simulink model "UnitTest_relay_model"  (Simulink 8.1)
settings: Solver=ode1  StartTime=0.0  StopTime=inf  FixedStep=Ts  MaxStep=1e-3  RelTol=1e-3
model workspace (MAT data in the model file):
  op_snapshot1 : opcond.OperatingPoint (value not decoded)
PostLoadFcn:
  | UnitTest_relay_model_init;
InitFcn:
  | UnitTest_relay_model_init;
values from neighbouring files (symbols this model uses):
  relay_par = xlsread('relay_parameters.xlsx')    [relay_settings_init.m]
undefined symbols (not defined in the file or in its folder): Ts
libraries: powerlib x3, rtlab x2, cables_lib x2, breaker_lib x2, artemis x1, simulink x1, relay_modbus_lib x1, rtio_generic_modbus x1, Load_lib x1, transformer_lib x1
settings Model: ARTEMISmethode_block_infos=$$__separator__$$UnitTest_relay_model/ARTEMIS Guide$$__separator__$$  Creator=RE25624  LastModifiedBy=re25624  BufferReuse=off
settings SolverCC: ZeroCrossAlgorithm=Adaptive
settings DataIOCC: ExternalInput=getinputstruct(op_snapshot1)  InitialState=getstatestruct(op_snapshot1)  LimitDataPoints=off  MaxDataPoints=90060  SignalLoggingSaveFormat=Dataset  SaveOutput=off  SignalLogging=off  DSMLogging=off  SaveTime=off  OutputSaveName=result
settings OptimizationCC: BlockReduction=off  OptimizeBlockIOStorage=off  BufferReuse=off  ExpressionFolding=off  LocalBlockOutputs=off
settings DebuggingCC: MaxConsecutiveZCsMsg=warning  IgnoredZcDiagnostic=none  SolverPrmCheckMsg=none  MultiTaskRateTransMsg=warning  FcnCallInpInsideContextMsg=EnableAllAsWarning  FrameProcessingCompatibilityMsg=error  ModelReferenceExtraNoncontSigs=warning  StrictBusMsg=None
settings ModelReferenceCC: UpdateModelReferenceTargets=IfOutOfDate
settings SFSimCC: SFSimEcho=off
settings GRTTargetCC: CodeReplacementLibrary=C89/C90 (ANSI)

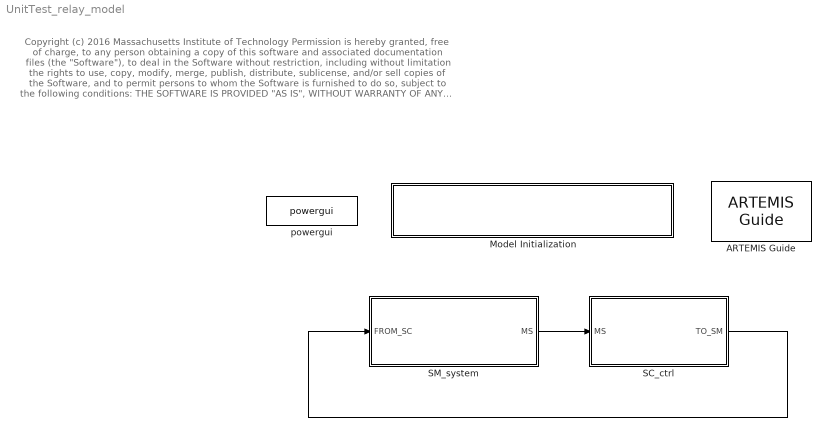
== system UnitTest_relay_model ==
  note: Copyright (c) 2016 Massachusetts Institute of Technology
      | Permission is hereby granted, free of charge, to any person obtaining a copy of this software and associated documentation files (the "Software"), to deal
      | in the Software without restriction, including without limitation the rights to use, copy, modify, merge, publish, distribute, sublicense, and/or sell copies of the
      | Software, and to permit persons to whom the Software is furnished to do so, subject to the following conditions:
      |
      | THE SOFTWARE IS PROVIDED "AS IS", WITHOUT WARRANTY OF ANY KIND, EXPRESS OR IMPLIED, INCLUDING BUT NOT LIMITED TO THE
      | WARRANTIES OF MERCHANTABILITY, FITNESS FOR A PARTICULAR PURPOSE AND NONINFRINGEMENT. IN NO EVENT SHALL THE AUTHORS
      | OR COPYRIGHT HOLDERS BE LIABLE FOR ANY CLAIM, DAMAGES OR OTHER LIABILITY, WHETHER IN AN ACTION OF CONTRACT, TORT OR
      | OTHERWISE, ARISING FROM, OUT OF OR IN CONNECTION WITH THE SOFTWARE OR THE USE OR OTHER DEALINGS IN THE SOFTWARE.
  ARTEMIS Guide : artemis/ARTEMIS/ARTEMIS Guide  Tag=FTSSmethode_opal_4hx0r99  Description=5.0_z1  lock=on  Ts=Ts  opt=art5  dyna=off  nb_perm=4  RT_fullcomp=off  ssn=on  ssn_itvc=off  ssn_ivic=off  ssn_ext=off  ssn_solver=Art5 with Backward Euler nodal interface  ssn_impulse=off  ssn_quasimpulse=off  ssn_impulse_loop=2  paraExtinctionThy=off  Thy_Impulse=on  dtc=Off  dtc_opt=normal  ao=on  simtype=off  ct_mac=off  lin_mov=off  lsp=[0.001 2]  spike_skip=Disabled  dtc_extra=1  dtc_sws=normal  dtc_pied=0.5  SPSRulesBlock=SPSRules  tre=on  ctmm=off  LF=off  dpl_type=ARTEMiS DPL  rlc_type=off  custom_type=off  para=on  ssn_ImpulseLoopBlockedStateUpdate=2  ssn_mov_iter_number=5  ssn_switch_iter_number=5
  Model Initialization : Subsystem  AncestorBlock=artemis/Tools /Misc/Model Initialization  mask(Model Functions){InitFcnX=UnitTest_relay_model_init;, prel=off, posl=on, inif=on, strf=off}
      mask prompts: InitFcnX "Initialisation"; prel "Preload Function"; posl "PostLoad Function"; inif "InitFcn"; strf "StartFcn"
      mask init:
      | currentBlock = gcb;
      | root = bdroot(currentBlock);
      | 
      | 
      | if ~strcmp(get_param(root,'BlockDiagramType'),'library')
      |     if prel==1
      |         set_param(root, 'PreLoadFcn', InitFcnX);
      |     else
      |         set_param(root, 'PreLoadFcn', '');
      |     end
      |     if inif==1
      |         set_param(root, 'InitFcn', InitFcnX);
      |     else
      |         set_param(root, 'InitFcn', '');
      |     end
      |     if strf==1
      |         set_param(root, 'StartFcn', InitFcnX);
      |     else
      |         set_param(root, 'StartFcn', '');
      |     end
      |     if posl==1
      |         set_param(root, 'PostLoadFcn', InitFcnX);
      |     else
      |         set_param(root, 'PostLoadFcn', '');
      |     end
      | end
      | 
      | pos = get_param(currentBlock, 'Position');
      | width = pos(3) - pos(1); height = pos(4) - pos(2);
      | txt = [ upper(root) '\n' '- InitFcn. . . . . '  get_param(root, 'InitFcn') ];
      settings: CopyFcn=set_param(gcb,'LinkStatus','inactive')
      mask Display: text(5, height*0.5, txt, 'horizontalAlignment', 'left', 'verticalAlignment', 'middle') ;
  SC_ctrl : Subsystem
  SM_system : Subsystem
  powergui : powerlib/powergui  Priority=2  SimulationMode=Discrete  SolverType=Tustin  SampleTime=Ts  frequency=60  SPID=off  DisableSnubberDevices=off  DisableRonSwitches=off  DisableVfSwitches=off  SwTol=0  Interpol=off  DisplayEquations=off  frequencyindice=0  Pbase=100e6  ErrMax=1e-4  Iterations=50  UnitsV=kV  UnitsW=MW  FunctionMessages=off  echomessages=off  HookPort=off  EnableUseOfTLC=off  x0status=blocks  RestoreLinks=warning  ResistiveCurrentMeasurement=off  Frange=logspace(0,3,50)  Ylog=off  Xlog=off  ShowGrid=off  save=off  variable=ZData  structure=0  ZoomFFT=on  StartTime=0.0  cycles=2  DisplayStyle=off  fundamental=60  FreqAxis=off  MaxFrequency=1000  frequencyindicesteady=1  RmsSteady=1  display=off  Ts=0  methode=off
  wires:
  SM_system/1(MS) -> SC_ctrl/1(MS)
  SC_ctrl/1(TO_SM) -> SM_system/1(FROM_SC)

== system UnitTest_relay_model/Model Initialization ==

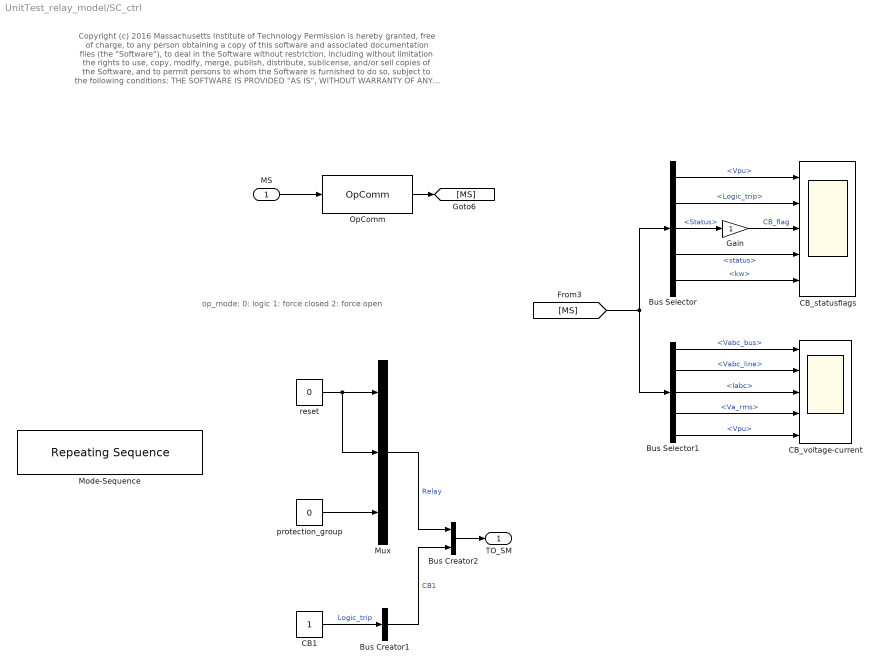
== system UnitTest_relay_model/SC_ctrl ==
  note: op_mode:
      | 0: logic
      | 1: force closed
      | 2: force open
  note: Copyright (c) 2016 Massachusetts Institute of Technology
      | Permission is hereby granted, free of charge, to any person obtaining a copy of this software and associated documentation files (the "Software"), to deal
      | in the Software without restriction, including without limitation the rights to use, copy, modify, merge, publish, distribute, sublicense, and/or sell copies of the
      | Software, and to permit persons to whom the Software is furnished to do so, subject to the following conditions:
      |
      | THE SOFTWARE IS PROVIDED "AS IS", WITHOUT WARRANTY OF ANY KIND, EXPRESS OR IMPLIED, INCLUDING BUT NOT LIMITED TO THE
      | WARRANTIES OF MERCHANTABILITY, FITNESS FOR A PARTICULAR PURPOSE AND NONINFRINGEMENT. IN NO EVENT SHALL THE AUTHORS
      | OR COPYRIGHT HOLDERS BE LIABLE FOR ANY CLAIM, DAMAGES OR OTHER LIABILITY, WHETHER IN AN ACTION OF CONTRACT, TORT OR
      | OTHERWISE, ARISING FROM, OUT OF OR IN CONNECTION WITH THE SOFTWARE OR THE USE OR OTHER DEALINGS IN THE SOFTWARE
  MS : Inport
  Bus Creator1 : BusCreator  Inputs=1
  Bus Creator2 : BusCreator  Inputs=2
  Bus Selector : BusSelector  OutputSignals=relay_cmd.m.Vpu,relay_cmd.Logic_trip,CB.Status,relay_cmd.m.status,relay_cmd.m.kw
  Bus Selector1 : BusSelector  OutputSignals=CB.Vabc_bus,CB.Vabc_line,CB.Iabc,relay_cmd.m.Va_rms,relay_cmd.m.Vpu
  CB1 : Constant
  CB_statusflags : Scope  NumInputPorts=5
      settings: ShowLegends=on  TimeRange=0.35  YMin=-0.01~-0.5~0~0~0  YMax=0.01~3~2~10~2500  SaveName=ScopeData6
  CB_voltage-current : Scope  NumInputPorts=5
      settings: ShowLegends=on  TimeRange=3  YMin=-12500~-12500~-175~0~0  YMax=12500~12500~175~10000~1.2
  Gain : Gain
  Mode-Sequence : simulink/Sources/Repeating Sequence  rep_seq_t=|  rep_seq_y=|
      rep_seq_t=|
      | [0
      | 2
      | 2
      | 4
      | 4
      | 6
      | 6
      | 8
      | 8
      | 10
      | 10
      | 12
      | 12
      | 14
      | 14
      | 16]
      rep_seq_y=|
      | [0
      | 0
      | 1
      | 1
      | 0
      | 0
      | 2
      | 2
      | 1
      | 1
      | 0
      | 0
      | 2
      | 2
      | 0
      | 0]
  Mux : Mux  Inputs=3
  OpComm : rtlab/OpComm  nbport=1  groupe_acq=1  subsys_rate=0  st=0  Synchronization=on  Interpolation=on  Threshold=1.0  Missed_Data=off  Sim_Time=off  Samples=off  dynSigOut=off  from_console=0  warning_done=off  writeOpCommFile=off  Offset=off
  protection_group : Constant  Value=0
  reset : Constant  Value=0
  TO_SM : Outport
  wires:
  OpComm/1 -> [MS]
  MS/1 -> OpComm/1
  [MS] -> Bus Selector/1, Bus Selector1/1
  Bus Selector/5 -> CB_statusflags/5  "<kw>"
  Bus Selector/1 -> CB_statusflags/1  "<Vpu>"
  Bus Selector/2 -> CB_statusflags/2  "<Logic_trip>"
  Bus Selector/4 -> CB_statusflags/4  "<status>"
  Bus Selector/3 -> Gain/1  "<Status>"
  Gain/1 -> CB_statusflags/3  "CB_flag"
  Bus Selector1/2 -> CB_voltage-current/2  "<Vabc_line>"
  Bus Selector1/1 -> CB_voltage-current/1  "<Vabc_bus>"
  Bus Selector1/3 -> CB_voltage-current/3  "<Iabc>"
  Mux/1 -> Bus Creator2/1  "Relay"
  reset/1 -> Mux/2, Mux/1
  protection_group/1 -> Mux/3
  Bus Selector1/4 -> CB_voltage-current/4  "<Va_rms>"
  Bus Selector1/5 -> CB_voltage-current/5  "<Vpu>"
  CB1/1 -> Bus Creator1/1  "Logic_trip"
  Bus Creator1/1 -> Bus Creator2/2  "CB1"
  Bus Creator2/1 -> TO_SM/1

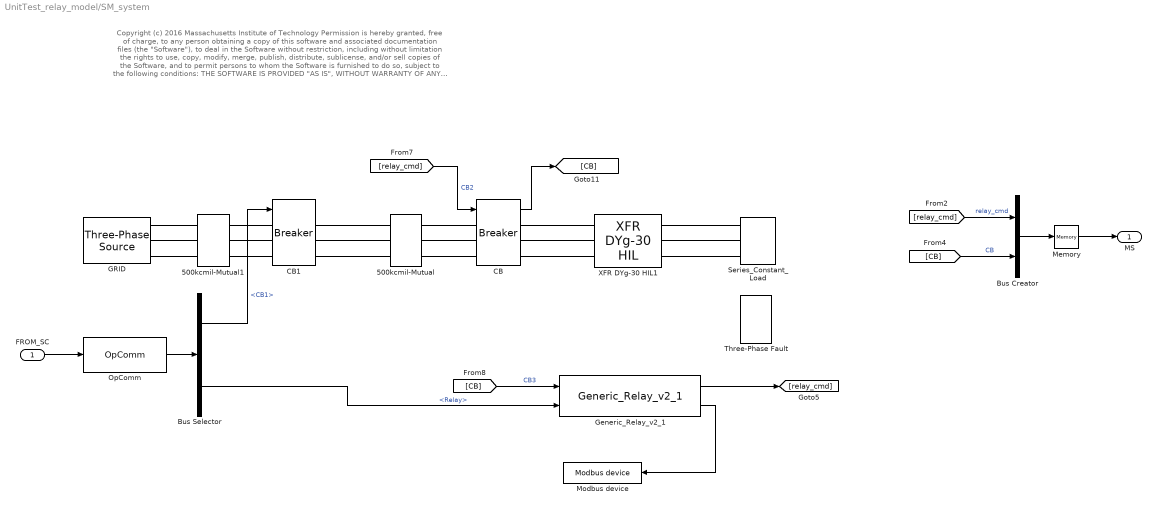
== system UnitTest_relay_model/SM_system ==
  note: Copyright (c) 2016 Massachusetts Institute of Technology
      | Permission is hereby granted, free of charge, to any person obtaining a copy of this software and associated documentation files (the "Software"), to deal
      | in the Software without restriction, including without limitation the rights to use, copy, modify, merge, publish, distribute, sublicense, and/or sell copies of the
      | Software, and to permit persons to whom the Software is furnished to do so, subject to the following conditions:
      |
      | THE SOFTWARE IS PROVIDED "AS IS", WITHOUT WARRANTY OF ANY KIND, EXPRESS OR IMPLIED, INCLUDING BUT NOT LIMITED TO THE
      | WARRANTIES OF MERCHANTABILITY, FITNESS FOR A PARTICULAR PURPOSE AND NONINFRINGEMENT. IN NO EVENT SHALL THE AUTHORS
      | OR COPYRIGHT HOLDERS BE LIABLE FOR ANY CLAIM, DAMAGES OR OTHER LIABILITY, WHETHER IN AN ACTION OF CONTRACT, TORT OR
      | OTHERWISE, ARISING FROM, OUT OF OR IN CONNECTION WITH THE SOFTWARE OR THE USE OR OTHER DEALINGS IN THE SOFTWARE
  FROM_SC : Inport
  500kcmil-Mutual : cables_lib/500kcmil-Mutual  length=1100  par_sets=1  ratio=3
  500kcmil-Mutual1 : cables_lib/500kcmil-Mutual  length=1100  par_sets=1  ratio=3
  Bus Creator : BusCreator  Inputs=2
  Bus Selector : BusSelector  OutputSignals=CB1,Relay
  CB : breaker_lib/Breaker  Ts=Ts  mech_delay=cb_mech_delay
  CB1 : breaker_lib/Breaker  Ts=Ts  mech_delay=cb_mech_delay
  GRID : powerlib/Electrical Sources/Three-Phase Source  Voltage=13800  PhaseAngle=0  Frequency=60  InternalConnection=Yg  SpecifyImpedance=on  Resistance=0.8929  Inductance=16.58e-3  ShortCircuitLevel=375e6  BaseVoltage=13800  XRratio=30  BusType=swing  Pref=0  Qref=0  Qmin=-inf  Qmax=inf
  Generic_Relay_v2_1 : relay_modbus_lib/Generic_Relay_v2_1  Ts=Ts  relay_settings=[relay_par(1,:)]
  Memory : Memory
  Modbus device : rtio_generic_modbus/Modbus device  conf_name=F1_relay_cfg2.opal  conf_name_mask=F1_relay_cfg2.xls  sample_time=Ts
  OpComm : rtlab/OpComm  nbport=1  groupe_acq=1  subsys_rate=0  st=0  Synchronization=on  Interpolation=on  Threshold=1.0  Missed_Data=off  Sim_Time=off  Samples=off  dynSigOut=off  from_console=1  warning_done=off  writeOpCommFile=off  Offset=off
  Series_Constant_Load : Load_lib/Series_Constant_Load  v=460  kVA=2500  pf=0.90
  Three-Phase Fault : powerlib/Elements/Three-Phase Fault  FaultA=on  FaultB=on  FaultC=on  FaultResistance=0.001  GroundFault=on  GroundResistance=0.001  External=off  SwitchStatus=[1 0]  SwitchTimes=[ 2.2 9]  InitialStates=[0 0 1]  SnubberResistance=1e6  SnubberCapacitance=inf  Measurements=None
  XFR DYg-30 HIL1 : transformer_lib/XFR DYg-30 HIL  Rating=2500  Vp=13800  Vs=480  Z=5.75  XR=6.6
  MS : Outport
  wires:
  CB/1 -> [CB]
  Bus Creator/1 -> Memory/1
  [relay_cmd] -> Bus Creator/1  "relay_cmd"
  [CB] -> Bus Creator/2  "CB"
  Memory/1 -> MS/1
  [CB] -> Generic_Relay_v2_1/1  "CB3"
  Generic_Relay_v2_1/1 -> [relay_cmd]
  [relay_cmd] -> CB/1  "CB2"
  Generic_Relay_v2_1/2 -> Modbus device/1
  FROM_SC/1 -> OpComm/1
  OpComm/1 -> Bus Selector/1
  Bus Selector/2 -> Generic_Relay_v2_1/2  "<Relay>"
  Bus Selector/1 -> CB1/1  "<CB1>"
  connections:
  500kcmil-Mutual/RConn2 -- CB/LConn2
  500kcmil-Mutual/RConn1 -- CB/LConn1
  500kcmil-Mutual/RConn3 -- CB/LConn3
  CB/RConn1 -- XFR DYg-30 HIL1/LConn1
  CB/RConn2 -- XFR DYg-30 HIL1/LConn2
  CB/RConn3 -- XFR DYg-30 HIL1/LConn3
  Series_Constant_Load/LConn2 -- XFR DYg-30 HIL1/RConn2
  Series_Constant_Load/LConn3 -- XFR DYg-30 HIL1/RConn3
  Series_Constant_Load/LConn1 -- XFR DYg-30 HIL1/RConn1
  500kcmil-Mutual/LConn2 -- CB1/RConn2
  500kcmil-Mutual/LConn1 -- CB1/RConn1
  500kcmil-Mutual/LConn3 -- CB1/RConn3
  500kcmil-Mutual1/RConn3 -- CB1/LConn3
  500kcmil-Mutual1/RConn2 -- CB1/LConn2
  500kcmil-Mutual1/RConn1 -- CB1/LConn1
  500kcmil-Mutual1/LConn2 -- GRID/RConn2
  500kcmil-Mutual1/LConn1 -- GRID/RConn1
  500kcmil-Mutual1/LConn3 -- GRID/RConn3
